simulink library "lib_supply_current_estimator"  (R2023a)
settings: Solver=VariableStepAuto  StartTime=0.0  StopTime=10.0  RelTol=1e-3
libraries: lib_conversion x1
settings Model: Creator=cav2ofo  LastModifiedBy=lenovo
settings OptimizationCC: ReuseModelBlockBuffer=off

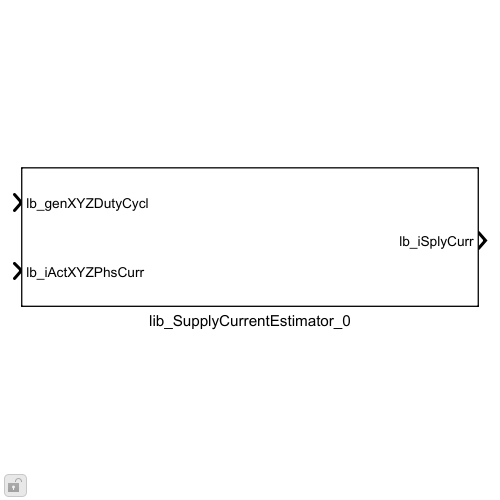
[thumbnail: Simulink's stored preview of the top-level diagram]
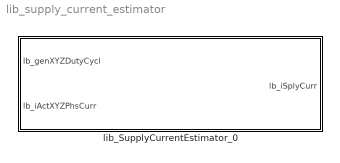
== system lib_supply_current_estimator ==
  lib_SupplyCurrentEstimator_0 : Subsystem  mask{lb_parOutpDataType=Inherit: Inherit via back propagation}
      mask prompts: lb_parOutpDataType "Output data type:"
      mask DialogControl DescGroupVar Prompt: VHIT control library
      mask DialogControl DescTextVar Prompt: Supply current estimator
      mask DialogControl ParameterGroupVar Prompt: Data type

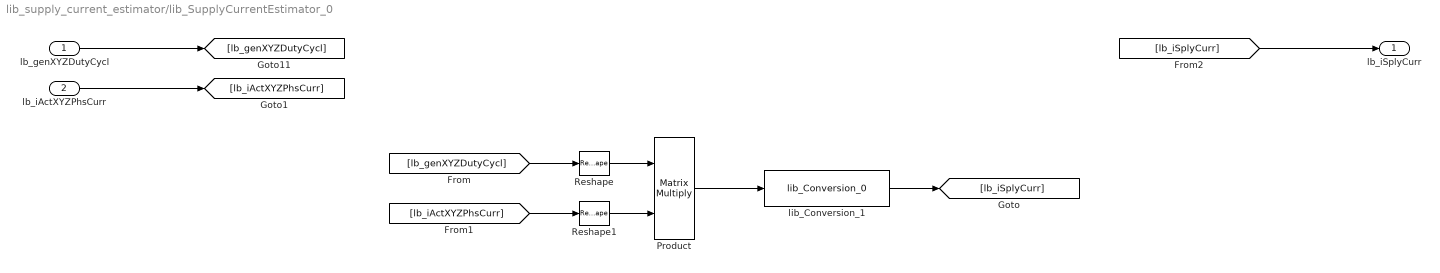
== system lib_supply_current_estimator/lib_SupplyCurrentEstimator_0 ==
  lb_genXYZDutyCycl : Inport
  lb_iActXYZPhsCurr : Inport  Port=2
  Product : Product  Multiplication=Matrix(*)  OutDataTypeStr=Inherit: Inherit via back propagation
  Reshape : Reshape  OutputDimensionality=Row vector (2-D)
  Reshape1 : Reshape  OutputDimensionality=Column vector (2-D)
  lib_Conversion_1 : lib_conversion/lib_Conversion_0  lb_parDataType=lb_parOutpDataType  lb_parOutpMaxVal=[]  lb_parOutpMinVal=[]  lb_parSatFlag=off
  lb_iSplyCurr : Outport
  wires:
  lb_genXYZDutyCycl/1 -> [lb_genXYZDutyCycl]
  lb_iActXYZPhsCurr/1 -> [lb_iActXYZPhsCurr]
  [lb_genXYZDutyCycl] -> Reshape/1
  [lb_iActXYZPhsCurr] -> Reshape1/1
  Reshape/1 -> Product/1
  Reshape1/1 -> Product/2
  Product/1 -> lib_Conversion_1/1
  [lb_iSplyCurr] -> lb_iSplyCurr/1
  lib_Conversion_1/1 -> [lb_iSplyCurr]
